simulink model "vg_proj"  (R2021b)
settings: Solver=FixedStepDiscrete  StartTime=0.0  StopTime=10.0  FixedStep=0.1  RelTol=1e-3  EnableMultiTasking=on
settings Model: Creator=anirudh  LastModifiedBy=anirudh
settings SolverCC: AlgebraicLoopSolver=TrustRegion  AutoInsertRateTranBlk=on
settings DataIOCC: LimitDataPoints=on
settings OptimizationCC: LifeSpan=inf
settings DebuggingCC: AllowSymbolicDim=off  SFUnexpectedBacktrackingDiag=warning  SFNoUnconditionalDefaultTransitionDiag=warning  SFExecutionAtInitializationDiag=none  ArithmeticOperatorsInVariantConditions=warning
settings SFSimCC: SimUseLocalCustomCode=off  CustomCodeUndefinedFunction=UseInterfaceOnly
settings RTWCC: RTWUseLocalCustomCode=off
settings CodeAppCC: StateflowObjectComments=on
settings GRTTargetCC: TargetLangStandard=C89/C90 (ANSI)
settings ConfigComp: CovMetricSettings=dw  CovSaveCumulativeToWorkspaceVar=on  CovSaveSingleToWorkspaceVar=on  CovExternalEMLEnable=off  CovSFcnEnable=off

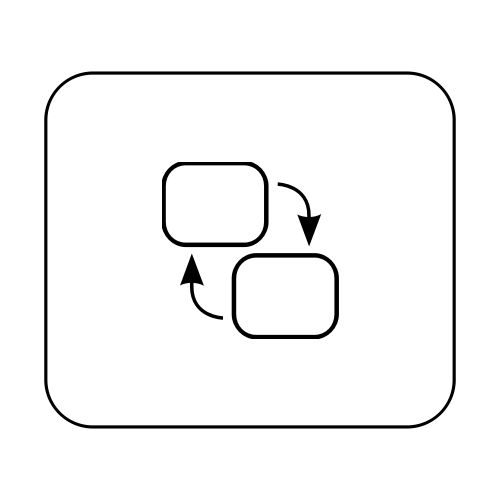
[thumbnail: Simulink's stored preview of the top-level diagram]
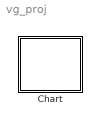
== system vg_proj ==
  Chart : Stateflow chart  TreatAsAtomicUnit=on

== stateflow chart vg_proj/Chart ==
  state Init
  state Inp_checker
    entry: inp = get_input();
  state Adv_checker
    entry: adv=check_adv();
    after(3,sec);
  state Stop
  Adv_checker -> Init [order 2] : [adv==0]
  Inp_checker -> Init [order 2] : [inp==0]
  Adv_checker -> Adv_checker [order 3] : [adv==2]
  (default) -> Init
  Init -> Inp_checker : after(3,sec)
  Inp_checker -> Adv_checker [order 1] : [inp==1]
  Adv_checker -> Stop [order 1] : [adv==1]
  data: adv local; inp local
